simulink model "STMF4Hall"  (R2024a)
settings: Solver=FixedStepAuto  StartTime=0.0  StopTime=inf  RelTol=1e-3  EnableMultiTasking=on
libraries: stm32f4xxblockslib x14, mcbpositiondecoderlib x4, stm32blockslib x2
settings Model: ExtModeTrigDuration=10  Creator=wsl  LastModifiedBy=wsl
settings SolverCC: AutoInsertRateTranBlk=on
settings OptimizationCC: EnhancedBackFolding=on  PassReuseOutputArgsAs=Individual arguments  ZeroExternalMemoryAtStartup=off  ZeroInternalMemoryAtStartup=off  MaxStackSize=64  OptimizeBlockOrder=speed  DifferentSizesBufferReuse=on  OptimizationCustomize=off  EfficientTunableParamExpr=on
settings DebuggingCC: MultiTaskDSMMsg=none  ParameterTunabilityLossMsg=error
settings HardwareCC: ProdBitPerPointer=32  ProdBitPerSizeT=32  ProdBitPerPtrDiffT=32  ProdLargestAtomicInteger=Long  ProdLargestAtomicFloat=Double  ProdWordSize=32  ProdLongLongMode=on  ProdHWDeviceType=ARM Compatible->ARM Cortex-M
settings SFSimCC: MATLABDynamicMemAlloc=off
settings RTWCC: Description=Embedded Coder  SystemTargetFile=ert.tlc  HardwareBoard=STM32F4xx Based  TemplateMakefile=ert_default_tmf  Toolchain=GNU Tools for ARM Embedded Processors
settings CodeAppCC: ForceParamTrailComments=on  IgnoreCustomStorageClasses=off  OperatorAnnotations=on  SimulinkDataObjDesc=on  SFDataObjDesc=on  InsertBlockDesc=on
settings ERTTargetCC: TargetLangStandard=C99 (ISO)  CodeReplacementLibrary=ARM Cortex-M  ExtModeTransport=3  ExtModeStaticAlloc=on  ExtModeStaticAllocSize=2048  ExtModeMexFile=ext_xcp  ExtModeIntrfLevel=Level2 - Open

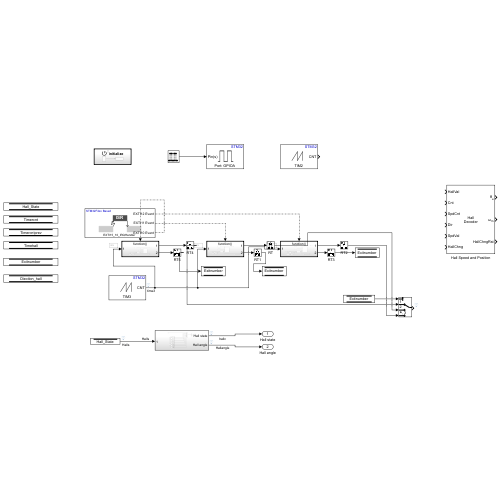
[thumbnail: Simulink's stored preview of the top-level diagram]
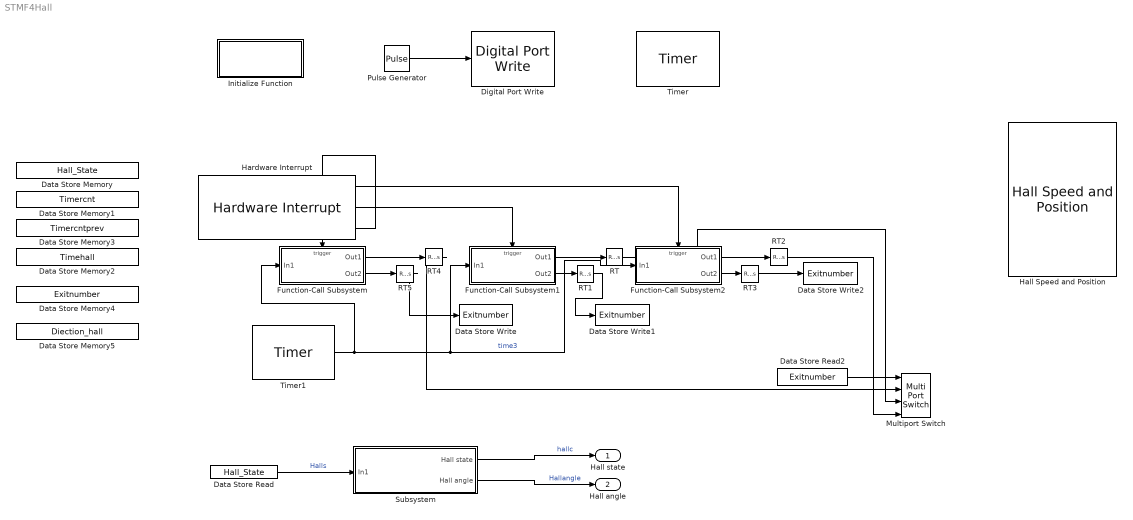
== system STMF4Hall ==
  Data Store Memory : DataStoreMemory  DataStoreName=Hall_State  WriteAfterWriteMsg=warning  ShowAdditionalParam=off
  Data Store Memory1 : DataStoreMemory  DataStoreName=Timercnt  WriteAfterWriteMsg=warning  ShowAdditionalParam=off
  Data Store Memory2 : DataStoreMemory  DataStoreName=Timehall  WriteAfterWriteMsg=warning  ShowAdditionalParam=off
  Data Store Memory3 : DataStoreMemory  DataStoreName=Timercntprev  WriteAfterWriteMsg=warning  ShowAdditionalParam=off
  Data Store Memory4 : DataStoreMemory  DataStoreName=Exitnumber  WriteAfterWriteMsg=warning  ShowAdditionalParam=off
  Data Store Memory5 : DataStoreMemory  DataStoreName=Diection_hall  WriteAfterWriteMsg=warning  ShowAdditionalParam=off
  Data Store Read : DataStoreRead  DataStoreName=Hall_State  IndexOptions=Index vector (dialog)  Indices=1  OutputSizes=1
  Data Store Read2 : DataStoreRead  DataStoreName=Exitnumber  IndexOptions=Index vector (dialog)  Indices=1  OutputSizes=1
  Data Store Write : DataStoreWrite  DataStoreName=Exitnumber  IndexOptions=Index vector (dialog)  Indices=1  OutputSizes=1
  Data Store Write1 : DataStoreWrite  DataStoreName=Exitnumber  IndexOptions=Index vector (dialog)  Indices=1  OutputSizes=1
  Data Store Write2 : DataStoreWrite  DataStoreName=Exitnumber  IndexOptions=Index vector (dialog)  Indices=1  OutputSizes=1
  Digital Port Write : stm32f4xxblockslib/Digital Port Write  PortName=GPIOA  PinNumber=[5]  ReadOperation=off  IOAsArray=on  EnableSimPort=off
  Function-Call Subsystem : Subsystem  TreatAsAtomicUnit=on
  Function-Call Subsystem1 : Subsystem  TreatAsAtomicUnit=on
  Function-Call Subsystem2 : Subsystem  TreatAsAtomicUnit=on
  Hall Speed and Position : mcbpositiondecoderlib/Hall Speed and Position  blkExecutionType=Speed and position  CounterSize=32 bits  ClkFreq=90e6  BlkSampleTime=50e-6  PolePairs=4  MinSpeed=20  HallInterruptConfig=Every 180 Degrees  SpeedUnit=RPM  PerUnitSpeed=1000  SpeedDataType=single  hallSequence=ABC  Sequence=[5,4,6,2,3,1]  EnableSecondOrder=1st Order  PositionUnit=Radians  PositionDataType=single
      settings: LibrarySourceBlock=mcblib/Sensor Decoders/Hall Speed and Position
  Hardware Interrupt : stm32f4xxblockslib/Hardware Interrupt  ISRGroup=External interrupts (EXTI)  ISRName=EXTI15_10_IRQHandler  ISRNumber=55  EventsList={ 'off', 'EXTI15 Event', '1'; 'off', 'EXTI14 Event', '2'; 'off', 'EXTI13 Event', '3'; 'on', 'EXTI12 Event', '4'; 'on', 'EXTI11 Event', '5'; 'on', 'EXTI10 Event', '6'; 'off', 'Custom event', '7' }  SelectedEvents={'EXTI12 Event','EXTI11 Event','EXTI10 Event'}  TaskPriority=30  DisablePreemption=on  ClearInterruptFlagsAtEndOfEvent=off  InterruptDefinitionFile=$(TARGET_ROOT)/registry/interrupts/STM32F4xxBased_interrupts.xml  HardwareBoard=STM32F4xx Based  EnableSimPort=off
  Initialize Function : Subsystem  TreatAsAtomicUnit=on
  Multiport Switch : MultiPortSwitch  SaturateOnIntegerOverflow=off  InputSameDT=off
  Pulse Generator : DiscretePulseGenerator  Period=10  PulseWidth=5  SampleTime=0.1
  RT{,1..5} (6 alike) : RateTransition  Deterministic=off  OutPortSampleTime=5e-05
  Subsystem : Subsystem
  Timer : stm32blockslib/Timer  TimerModule=TIM2  EnableFrequencyInput=off  EnableCounterInput=off  EnableMainOutputInput=off  SetRCAfterCE=off  OutputDirection=off  OutputMainOutputEnableStatus=off  SampleTime=-1  EnableUpdateEvent=off  EnableCaptureCompare1Event=off  EnableCaptureCompare2Event=off  EnableCaptureCompare3Event=off  EnableCaptureCompare4Event=off  EnableTriggerEvent=off  EnableBreakEvent=off  EnableBreakEvent2=off  EnableCOMGenerationEvent=off  ProcessorFamily=STM32F7
      settings: LibrarySourceBlock=stm32f4xxblockslib/Timer
  Timer1 : stm32blockslib/Timer  TimerModule=TIM3  EnableFrequencyInput=off  EnableCounterInput=off  EnableMainOutputInput=off  SetRCAfterCE=off  OutputDirection=off  OutputMainOutputEnableStatus=off  SampleTime=-1  EnableUpdateEvent=off  EnableCaptureCompare1Event=off  EnableCaptureCompare2Event=off  EnableCaptureCompare3Event=off  EnableCaptureCompare4Event=off  EnableTriggerEvent=off  EnableBreakEvent=off  EnableBreakEvent2=off  EnableCOMGenerationEvent=off  ProcessorFamily=STM32F7
      settings: LibrarySourceBlock=stm32f4xxblockslib/Timer
  Hall state : Outport
  Hall angle : Outport  Port=2
  wires:
  Pulse Generator/1 -> Digital Port Write/1
  Hardware Interrupt/3 -> Function-Call Subsystem/Trigger
  Hardware Interrupt/2 -> Function-Call Subsystem1/Trigger
  Hardware Interrupt/1 -> Function-Call Subsystem2/Trigger
  Data Store Read/1 -> Subsystem/1(In1)  "Halls"
  Subsystem/1(Hall state) -> Hall state/1  "hallc"
  Subsystem/2(Hall angle) -> Hall angle/1  "Hallangle"
  Timer1/1 -> Function-Call Subsystem2/1(In1), Function-Call Subsystem1/1(In1), Function-Call Subsystem/1(In1)  "time3"
  RT5/1 -> Data Store Write/1
  RT1/1 -> Data Store Write1/1
  RT3/1 -> Data Store Write2/1
  Data Store Read2/1 -> Multiport Switch/1
  RT4/1 -> Multiport Switch/2
  RT/1 -> Multiport Switch/3
  RT2/1 -> Multiport Switch/4
  Function-Call Subsystem1/1(Out1) -> RT/1
  Function-Call Subsystem1/2(Out2) -> RT1/1
  Function-Call Subsystem2/1(Out1) -> RT2/1
  Function-Call Subsystem2/2(Out2) -> RT3/1
  Function-Call Subsystem/1(Out1) -> RT4/1
  Function-Call Subsystem/2(Out2) -> RT5/1

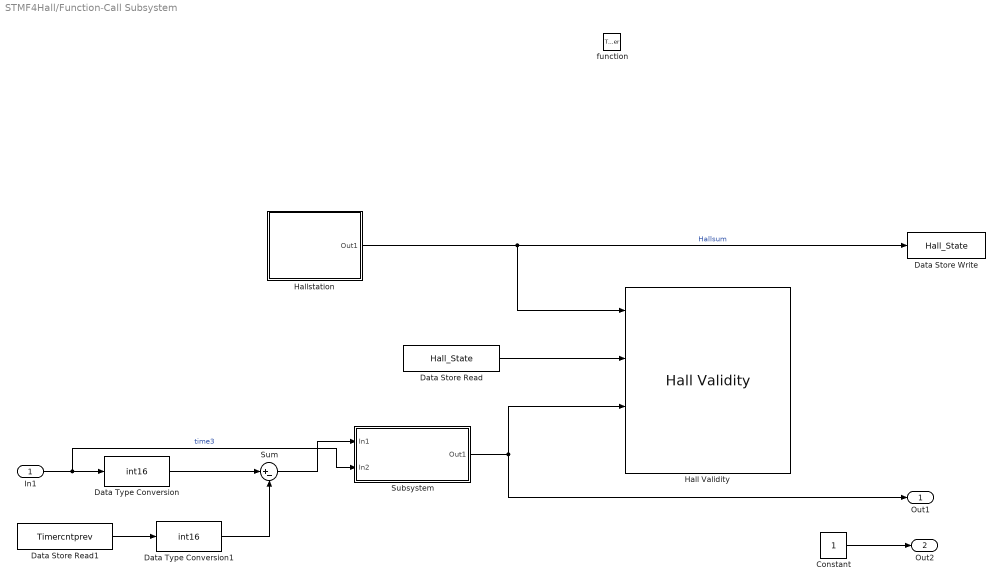
== system STMF4Hall/Function-Call Subsystem ==
  In1 : Inport
  function : TriggerPort  TriggerType=function-call  VariantControl=(inherit)
  Constant : Constant
  Data Store Read : DataStoreRead  DataStoreName=Hall_State  IndexOptions=Index vector (dialog)  Indices=1  OutputSizes=1
  Data Store Read1 : DataStoreRead  DataStoreName=Timercntprev  IndexOptions=Index vector (dialog)  Indices=1  OutputSizes=1
  Data Store Write : DataStoreWrite  DataStoreName=Hall_State  IndexOptions=Index vector (dialog)  Indices=1  OutputSizes=1
  Data Type Conversion : DataTypeConversion  OutDataTypeStr=int16  SaturateOnIntegerOverflow=off  RndMeth=Floor
  Data Type Conversion1 : DataTypeConversion  OutDataTypeStr=int16  SaturateOnIntegerOverflow=off  RndMeth=Floor
  Hall Validity : mcbpositiondecoderlib/Hall Validity  hallSequence=ABC  sequence=[5,4,6,2,3,1]  CounterSize=16 bits
  Hallstation : Subsystem
  Subsystem : Subsystem
  Sum : Sum  Inputs=|+-
  Out1 : Outport
  Out2 : Outport  Port=2
  wires:
  Hallstation/1(Out1) -> Hall Validity/1, Data Store Write/1  "Hallsum"
  Data Store Read/1 -> Hall Validity/2
  In1/1 -> Subsystem/2(In2), Data Type Conversion/1  "time3"
  Data Type Conversion/1 -> Sum/1
  Data Store Read1/1 -> Data Type Conversion1/1
  Sum/1 -> Subsystem/1(In1)
  Data Type Conversion1/1 -> Sum/2
  Subsystem/1(Out1) -> Hall Validity/3, Out1/1
  Constant/1 -> Out2/1

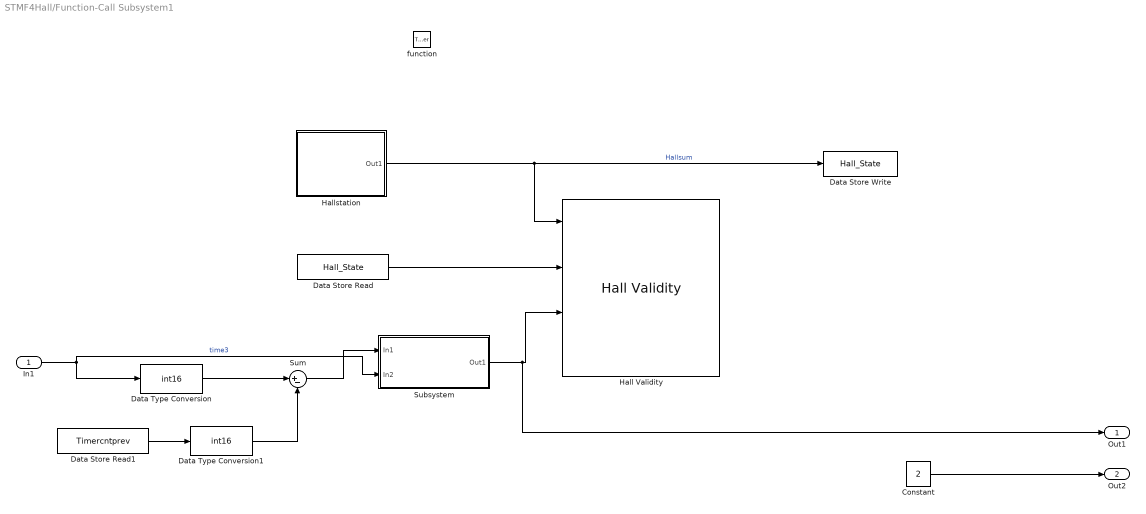
== system STMF4Hall/Function-Call Subsystem1 ==
  In1 : Inport
  function : TriggerPort  TriggerType=function-call  VariantControl=(inherit)
  Constant : Constant  Value=2
  Data Store Read : DataStoreRead  DataStoreName=Hall_State  IndexOptions=Index vector (dialog)  Indices=1  OutputSizes=1
  Data Store Read1 : DataStoreRead  DataStoreName=Timercntprev  IndexOptions=Index vector (dialog)  Indices=1  OutputSizes=1
  Data Store Write : DataStoreWrite  DataStoreName=Hall_State  IndexOptions=Index vector (dialog)  Indices=1  OutputSizes=1
  Data Type Conversion : DataTypeConversion  OutDataTypeStr=int16  SaturateOnIntegerOverflow=off  RndMeth=Floor
  Data Type Conversion1 : DataTypeConversion  OutDataTypeStr=int16  SaturateOnIntegerOverflow=off  RndMeth=Floor
  Hall Validity : mcbpositiondecoderlib/Hall Validity  hallSequence=ABC  sequence=[5,4,6,2,3,1]  CounterSize=16 bits
  Hallstation : Subsystem
  Subsystem : Subsystem
  Sum : Sum  Inputs=|+-
  Out1 : Outport
  Out2 : Outport  Port=2
  wires:
  Subsystem/1(Out1) -> Out1/1, Hall Validity/3
  Data Type Conversion1/1 -> Sum/2
  Sum/1 -> Subsystem/1(In1)
  In1/1 -> Data Type Conversion/1, Subsystem/2(In2)  "time3"
  Data Store Read1/1 -> Data Type Conversion1/1
  Hallstation/1(Out1) -> Hall Validity/1, Data Store Write/1  "Hallsum"
  Data Store Read/1 -> Hall Validity/2
  Data Type Conversion/1 -> Sum/1
  Constant/1 -> Out2/1

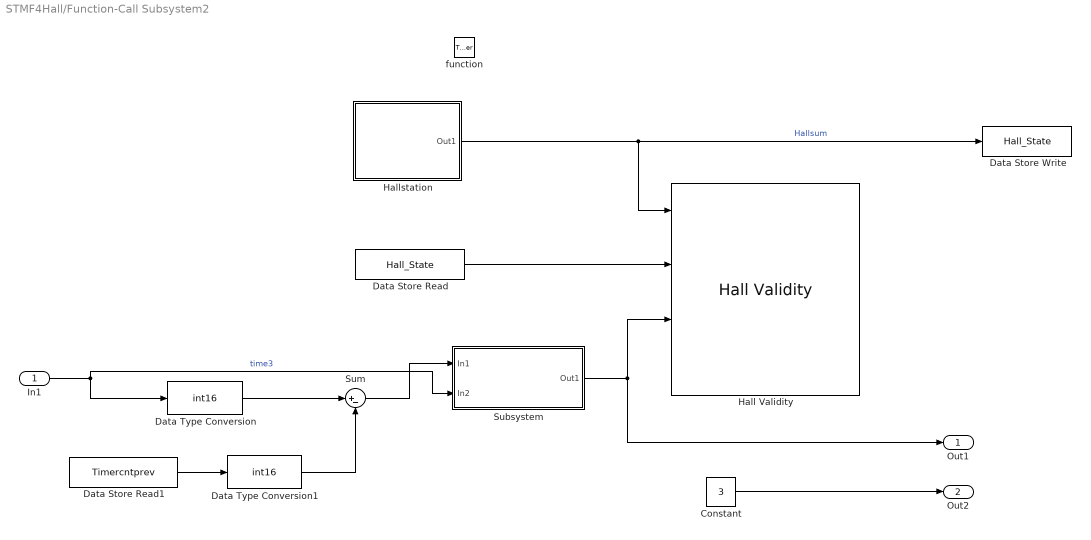
== system STMF4Hall/Function-Call Subsystem2 ==
  In1 : Inport
  function : TriggerPort  TriggerType=function-call  VariantControl=(inherit)
  Constant : Constant  Value=3
  Data Store Read : DataStoreRead  DataStoreName=Hall_State  IndexOptions=Index vector (dialog)  Indices=1  OutputSizes=1
  Data Store Read1 : DataStoreRead  DataStoreName=Timercntprev  IndexOptions=Index vector (dialog)  Indices=1  OutputSizes=1
  Data Store Write : DataStoreWrite  DataStoreName=Hall_State  IndexOptions=Index vector (dialog)  Indices=1  OutputSizes=1
  Data Type Conversion : DataTypeConversion  OutDataTypeStr=int16  SaturateOnIntegerOverflow=off  RndMeth=Floor
  Data Type Conversion1 : DataTypeConversion  OutDataTypeStr=int16  SaturateOnIntegerOverflow=off  RndMeth=Floor
  Hall Validity : mcbpositiondecoderlib/Hall Validity  hallSequence=ABC  sequence=[5,4,6,2,3,1]  CounterSize=16 bits
  Hallstation : Subsystem
  Subsystem : Subsystem
  Sum : Sum  Inputs=|+-
  Out1 : Outport
  Out2 : Outport  Port=2
  wires:
  In1/1 -> Data Type Conversion/1, Subsystem/2(In2)  "time3"
  Data Type Conversion/1 -> Sum/1
  Hallstation/1(Out1) -> Hall Validity/1, Data Store Write/1  "Hallsum"
  Data Store Read1/1 -> Data Type Conversion1/1
  Sum/1 -> Subsystem/1(In1)
  Subsystem/1(Out1) -> Hall Validity/3, Out1/1
  Data Type Conversion1/1 -> Sum/2
  Data Store Read/1 -> Hall Validity/2
  Constant/1 -> Out2/1

== system STMF4Hall/Initialize Function ==
  Data Store Write : DataStoreWrite  DataStoreName=Hall_State  IndexOptions=Index vector (dialog)  Indices=1  OutputSizes=1
  Event Listener : EventListener  DisableCoverage=on  EventName=reset
  Hallstation : Subsystem
  wires:
  Hallstation/1(Out1) -> Data Store Write/1

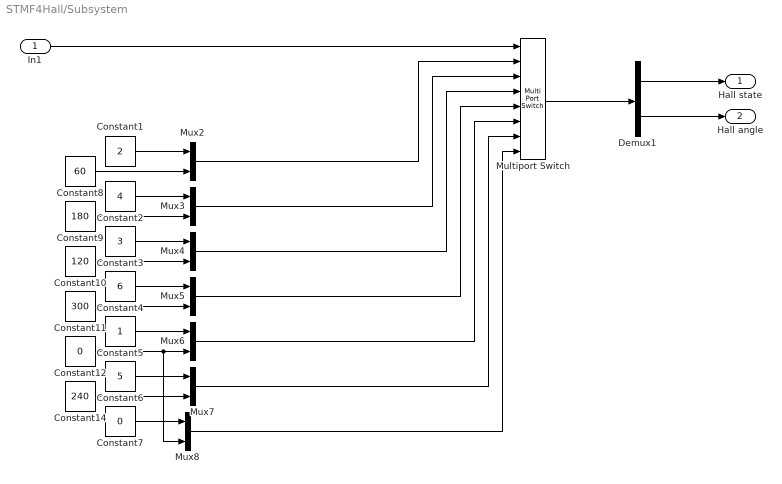
== system STMF4Hall/Subsystem ==
  In1 : Inport
  Constant1 : Constant  Value=2
  Constant10 : Constant  Value=120
  Constant11 : Constant  Value=300
  Constant12 : Constant  Value=0
  Constant14 : Constant  Value=240
  Constant2 : Constant  Value=4
  Constant3 : Constant  Value=3
  Constant4 : Constant  Value=6
  Constant5 : Constant
  Constant6 : Constant  Value=5
  Constant7 : Constant  Value=0
  Constant8 : Constant  Value=60
  Constant9 : Constant  Value=180
  Demux1 : Demux  Outputs=2
  Multiport Switch : MultiPortSwitch  Inputs=6  DataPortForDefault=Additional data port  SaturateOnIntegerOverflow=off  InputSameDT=off
  Mux{2..8} (7 alike) : Mux  Inputs=2
  Hall state : Outport
  Hall angle : Outport  Port=2
  wires:
  Demux1/2 -> Hall angle/1
  Constant8/1 -> Mux2/2
  Mux7/1 -> Multiport Switch/7
  Constant11/1 -> Mux5/2
  Mux6/1 -> Multiport Switch/6
  Constant5/1 -> Mux6/1
  Multiport Switch/1 -> Demux1/1
  Constant3/1 -> Mux4/1
  Constant4/1 -> Mux5/1
  Constant1/1 -> Mux2/1
  Constant10/1 -> Mux4/2
  Constant2/1 -> Mux3/1
  Demux1/1 -> Hall state/1
  Constant12/1 -> Mux8/2, Mux6/2
  Constant14/1 -> Mux7/2
  Constant9/1 -> Mux3/2
  Mux2/1 -> Multiport Switch/2
  Mux8/1 -> Multiport Switch/8
  Constant6/1 -> Mux7/1
  Constant7/1 -> Mux8/1
  Mux3/1 -> Multiport Switch/3
  Mux4/1 -> Multiport Switch/4
  Mux5/1 -> Multiport Switch/5
  In1/1 -> Multiport Switch/1

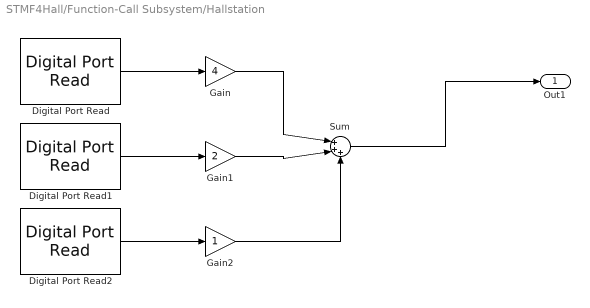
== system STMF4Hall/Function-Call Subsystem/Hallstation ==
  Digital Port Read : stm32f4xxblockslib/Digital Port Read  PortName=GPIOC  PinNumber=[10]  ReadOperation=on  IOAsArray=on  SampleTime=-1  EnableSimPort=off
  Digital Port Read1 : stm32f4xxblockslib/Digital Port Read  PortName=GPIOC  PinNumber=[11]  ReadOperation=on  IOAsArray=on  SampleTime=-1  EnableSimPort=off
  Digital Port Read2 : stm32f4xxblockslib/Digital Port Read  PortName=GPIOC  PinNumber=[12]  ReadOperation=on  IOAsArray=on  SampleTime=-1  EnableSimPort=off
  Gain : Gain  Gain=4  OutDataTypeStr=uint8
  Gain1 : Gain  Gain=2  OutDataTypeStr=uint8
  Gain2 : Gain  OutDataTypeStr=uint8
  Sum : Sum  Inputs=|+++
  Out1 : Outport
  wires:
  Digital Port Read1/1 -> Gain1/1
  Digital Port Read2/1 -> Gain2/1
  Digital Port Read/1 -> Gain/1
  Gain2/1 -> Sum/3
  Gain1/1 -> Sum/2
  Gain/1 -> Sum/1
  Sum/1 -> Out1/1

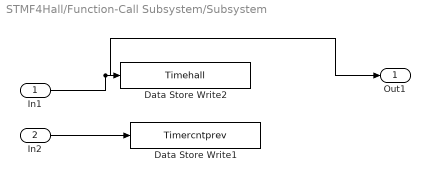
== system STMF4Hall/Function-Call Subsystem/Subsystem ==
  In1 : Inport
  In2 : Inport  Port=2
  Data Store Write1 : DataStoreWrite  DataStoreName=Timercntprev  IndexOptions=Index vector (dialog)  Indices=1  OutputSizes=1
  Data Store Write2 : DataStoreWrite  DataStoreName=Timehall  IndexOptions=Index vector (dialog)  Indices=1  OutputSizes=1
  Out1 : Outport
  wires:
  In1/1 -> Out1/1, Data Store Write2/1
  In2/1 -> Data Store Write1/1

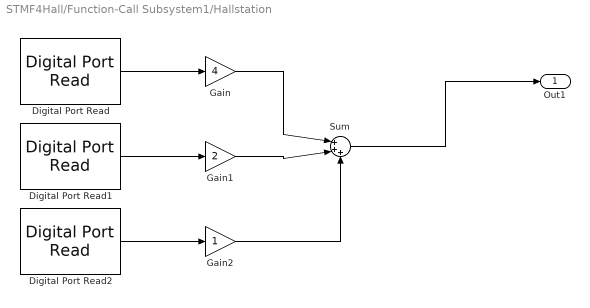
== system STMF4Hall/Function-Call Subsystem1/Hallstation ==
  Digital Port Read : stm32f4xxblockslib/Digital Port Read  PortName=GPIOC  PinNumber=[10]  ReadOperation=on  IOAsArray=on  SampleTime=-1  EnableSimPort=off
  Digital Port Read1 : stm32f4xxblockslib/Digital Port Read  PortName=GPIOC  PinNumber=[11]  ReadOperation=on  IOAsArray=on  SampleTime=-1  EnableSimPort=off
  Digital Port Read2 : stm32f4xxblockslib/Digital Port Read  PortName=GPIOC  PinNumber=[12]  ReadOperation=on  IOAsArray=on  SampleTime=-1  EnableSimPort=off
  Gain : Gain  Gain=4  OutDataTypeStr=uint8
  Gain1 : Gain  Gain=2  OutDataTypeStr=uint8
  Gain2 : Gain  OutDataTypeStr=uint8
  Sum : Sum  Inputs=|+++
  Out1 : Outport
  wires:
  Digital Port Read1/1 -> Gain1/1
  Digital Port Read2/1 -> Gain2/1
  Digital Port Read/1 -> Gain/1
  Gain2/1 -> Sum/3
  Gain1/1 -> Sum/2
  Gain/1 -> Sum/1
  Sum/1 -> Out1/1

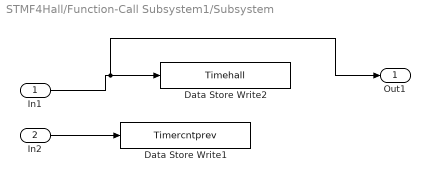
== system STMF4Hall/Function-Call Subsystem1/Subsystem ==
  In1 : Inport
  In2 : Inport  Port=2
  Data Store Write1 : DataStoreWrite  DataStoreName=Timercntprev  IndexOptions=Index vector (dialog)  Indices=1  OutputSizes=1
  Data Store Write2 : DataStoreWrite  DataStoreName=Timehall  IndexOptions=Index vector (dialog)  Indices=1  OutputSizes=1
  Out1 : Outport
  wires:
  In1/1 -> Out1/1, Data Store Write2/1
  In2/1 -> Data Store Write1/1

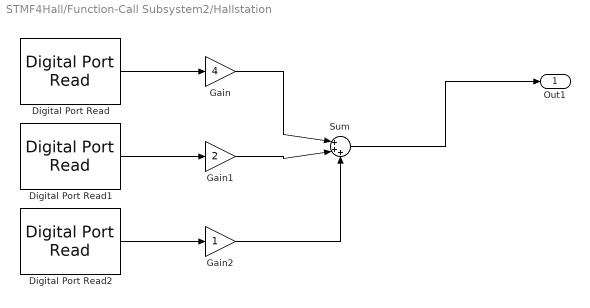
== system STMF4Hall/Function-Call Subsystem2/Hallstation ==
  Digital Port Read : stm32f4xxblockslib/Digital Port Read  PortName=GPIOC  PinNumber=[10]  ReadOperation=on  IOAsArray=on  SampleTime=-1  EnableSimPort=off
  Digital Port Read1 : stm32f4xxblockslib/Digital Port Read  PortName=GPIOC  PinNumber=[11]  ReadOperation=on  IOAsArray=on  SampleTime=-1  EnableSimPort=off
  Digital Port Read2 : stm32f4xxblockslib/Digital Port Read  PortName=GPIOC  PinNumber=[12]  ReadOperation=on  IOAsArray=on  SampleTime=-1  EnableSimPort=off
  Gain : Gain  Gain=4  OutDataTypeStr=uint8
  Gain1 : Gain  Gain=2  OutDataTypeStr=uint8
  Gain2 : Gain  OutDataTypeStr=uint8
  Sum : Sum  Inputs=|+++
  Out1 : Outport
  wires:
  Digital Port Read1/1 -> Gain1/1
  Digital Port Read2/1 -> Gain2/1
  Digital Port Read/1 -> Gain/1
  Gain2/1 -> Sum/3
  Gain1/1 -> Sum/2
  Gain/1 -> Sum/1
  Sum/1 -> Out1/1

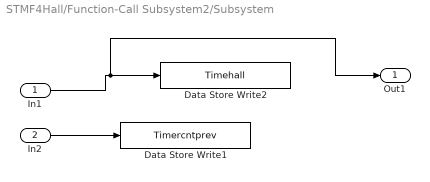
== system STMF4Hall/Function-Call Subsystem2/Subsystem ==
  In1 : Inport
  In2 : Inport  Port=2
  Data Store Write1 : DataStoreWrite  DataStoreName=Timercntprev  IndexOptions=Index vector (dialog)  Indices=1  OutputSizes=1
  Data Store Write2 : DataStoreWrite  DataStoreName=Timehall  IndexOptions=Index vector (dialog)  Indices=1  OutputSizes=1
  Out1 : Outport
  wires:
  In1/1 -> Out1/1, Data Store Write2/1
  In2/1 -> Data Store Write1/1

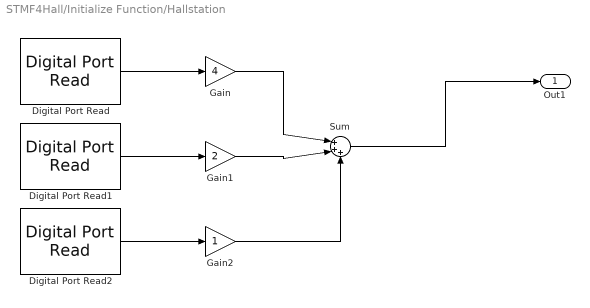
== system STMF4Hall/Initialize Function/Hallstation ==
  Digital Port Read : stm32f4xxblockslib/Digital Port Read  PortName=GPIOC  PinNumber=[10]  ReadOperation=on  IOAsArray=on  SampleTime=-1  EnableSimPort=off
  Digital Port Read1 : stm32f4xxblockslib/Digital Port Read  PortName=GPIOC  PinNumber=[11]  ReadOperation=on  IOAsArray=on  SampleTime=-1  EnableSimPort=off
  Digital Port Read2 : stm32f4xxblockslib/Digital Port Read  PortName=GPIOC  PinNumber=[12]  ReadOperation=on  IOAsArray=on  SampleTime=-1  EnableSimPort=off
  Gain : Gain  Gain=4  OutDataTypeStr=uint8
  Gain1 : Gain  Gain=2  OutDataTypeStr=uint8
  Gain2 : Gain  OutDataTypeStr=uint8
  Sum : Sum  Inputs=|+++
  Out1 : Outport
  wires:
  Digital Port Read1/1 -> Gain1/1
  Digital Port Read2/1 -> Gain2/1
  Digital Port Read/1 -> Gain/1
  Gain2/1 -> Sum/3
  Gain1/1 -> Sum/2
  Gain/1 -> Sum/1
  Sum/1 -> Out1/1
